simulink model "example_01"  (R2019b)
settings: Solver=VariableStepAuto  StartTime=0.0  StopTime=5680  RelTol=1e-12
libraries: DQ_SR_LIB_SIM x5, SAMPLE_systems x1
settings Model: Creator=AurelianoRivolta  LastModifiedBy=AurelianoRivolta

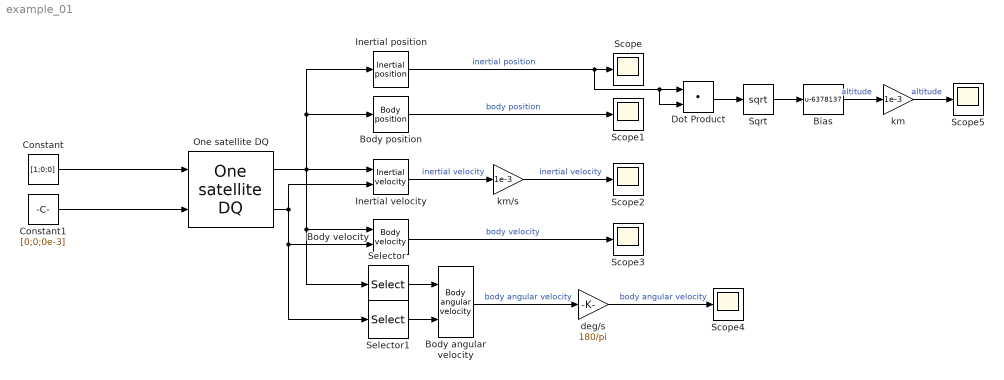
== system example_01 ==
  Bias : Bias  Bias=-6378137
  Body angular velocity : DQ_SR_LIB_SIM/Utilities/Body  angular velocity
  Body position : DQ_SR_LIB_SIM/Utilities/Body  position
  Body velocity : DQ_SR_LIB_SIM/Utilities/Body  velocity
  Constant : Constant  Value=[1;0;0]
  Constant1 : Constant  Value=[0;0;0e-3]
  Dot Product : DotProduct  InputSameDT=on  OutDataTypeStr=Inherit: Inherit via internal rule
  Inertial position : DQ_SR_LIB_SIM/Utilities/Inertial  position
  Inertial velocity : DQ_SR_LIB_SIM/Utilities/Inertial  velocity
  One satellite DQ : SAMPLE_systems/One satellite DQ  M=100  I=[20 30 40]'  a=6378137+500*1e3  ecc=0  incl=0  RAAN=0  omega=0  theta=0  q0=zq  omega_b=[0;0;1e-3]  isin=off
  Scope{,1..5} (6 alike) : Scope
  Selector : Selector  InputPortWidth=8  IndexOptions=Index vector (dialog)  Indices=1:4  OutputSizes=1
  Selector1 : Selector  InputPortWidth=8  IndexOptions=Index vector (dialog)  Indices=1:4  OutputSizes=1
  Sqrt : Sqrt  SaturateOnIntegerOverflow=on
  deg/s : Gain  Gain=180/pi
  km : Gain  Gain=1e-3
  km/s : Gain  Gain=1e-3
  wires:
  Constant/1 -> One satellite DQ/1
  Constant1/1 -> One satellite DQ/2
  One satellite DQ/2 -> Inertial velocity/2, Body velocity/2, Selector1/1
  Inertial position/1 -> Dot Product/2, Dot Product/1, Scope/1  "inertial position"
  Body position/1 -> Scope1/1  "body position"
  km/s/1 -> Scope2/1  "inertial velocity"
  Body velocity/1 -> Scope3/1  "body velocity"
  One satellite DQ/1 -> Inertial velocity/1, Body position/1, Inertial position/1, Body velocity/1, Selector/1
  Selector/1 -> Body angular velocity/1
  Selector1/1 -> Body angular velocity/2
  Body angular velocity/1 -> deg/s/1  "body angular velocity"
  Inertial velocity/1 -> km/s/1  "inertial velocity"
  Dot Product/1 -> Sqrt/1
  Sqrt/1 -> Bias/1
  km/1 -> Scope5/1  "altitude"
  Bias/1 -> km/1  "altitude"
  deg/s/1 -> Scope4/1  "body angular velocity"
